simulink model "Galvo_sys_Cdisc_Pcont_cc_nosub_GUT_v63_algebLoop_refMods_101114"  (R2013a)
settings: Solver=ode45  StartTime=0.0  StopTime=10e-3  FixedStep=FS  MaxStep=1e-4  RelTol=1e-3
PreLoadFcn:
  | vname=@(x) inputname(1);
  | paramCtrl=evalin('base','paramCtrl;');
  | I_LIM=str2num(paramCtrl.I_LIM);
  | Kbc=str2num(paramCtrl.Kbc);
  | FS=evalin('base','FS;');
InitFcn:
  | %%%%%%  set scope time range
  | T_STOP=str2num(get_param(gcs,'StopTime'));
  | if numel(T_STOP) > 1
  |    T_STOP=T_STOP(2);
  | else
  |    T_STOP=T_STOP(1);
  | end
  | T_STOP=num2str(T_STOP);
  | 
  | %%%%%%  set scope time range in system @init_callback_fct
  | T_STOP=num2str(str2num(get_param(gcs,'StopTime')));
  | 
  | childs = allchild(0);
  | sol=strfind(upper(get(allchild(0),'Tag')),'VIEWER_PARAMETERS');
  | 
  | if iscell(sol)
  |    ind=find(~cellfun(@isempty, strfind(upper(get(allchild(0),'Tag')),'VIEWER_PARAMETERS')));
  | else
  |    ind=sol;
  | end
  | %ind=find(~cellfun(@isempty, {strfind(upper(get(allchild(0),'Tag')),'VIEWER_PARAMETERS'),[]}))
  | if ~isempty(ind)
  |    for k=1:length(childs(ind))
  |       set_param(getfield(get(childs(ind(k)),'UserData'),'block'),'TimeRange',T_STOP);
  |       get_param(getfield(get(childs(ind(k)),'UserData'),'block'),'TimeRange');
  | %    set_param(getfield(get(childs(ind),'UserData'),'block'),'TimeRange',T_STOP);
  | %    get_param(getfield(get(childs(ind),'UserData'),'block'),'TimeRange');
  |    end
  | else
  |     warning(sprintf('VIEWER_PARAMETERS object not found\nOpen the config dialog by hand for the first sim start'))
  | end
StartFcn:
  | I_LIM=str2num(paramCtrl.I_LIM);
  | Kbc=str2num(paramCtrl.Kbc);
  | %FS=evalin('base','FS;');
values from neighbouring files (symbols this model uses):
  FB_EN = 1    [GalvoModel_v6_sys.m]    (also in Galvo_process_analyze.m = k-1; kompl_kreis_linmod_sensitiv.m)
  Lc = 170e-6    (= 0.00017)    [GalvoModel_v6_sys.m]    (also in Galvo_process_analyze.m)
  Rc = 1.5    [GalvoModel_v6_sys.m]    (also in Galvo_process_analyze.m; frequenzgang_nichtinvert_opamp_koblitz_eas.m = 1)
  Rsh = 0.003    [GalvoModel_v6_sys.m]    (also in Galvo_sys_proto_v13_OFFSETS_MODEL_PT1B_proc.m = 0.075; frequenzgang_nichtinvert_opamp_koblitz_eas.m = 0.015)
undefined symbols (not defined in the file or in its folder): JR, KBM, KFR, KMT, KTB
libraries: simulink x2, simulink_extras x1, dspsigops x1
settings Model: BufferReuse=off  Creator=mainster  LastModifiedBy=mainster
settings SolverCC: AutoInsertRateTranBlk=on
settings DataIOCC: LimitDataPoints=off  SaveOutput=off  SaveTime=off
settings OptimizationCC: BlockReduction=off  OptimizeBlockIOStorage=off  BufferReuse=off  ExpressionFolding=off  LocalBlockOutputs=off
settings ModelReferenceCC: ModelReferenceNumInstancesAllowed=Single  ModelReferenceMinAlgLoopOccurrences=on

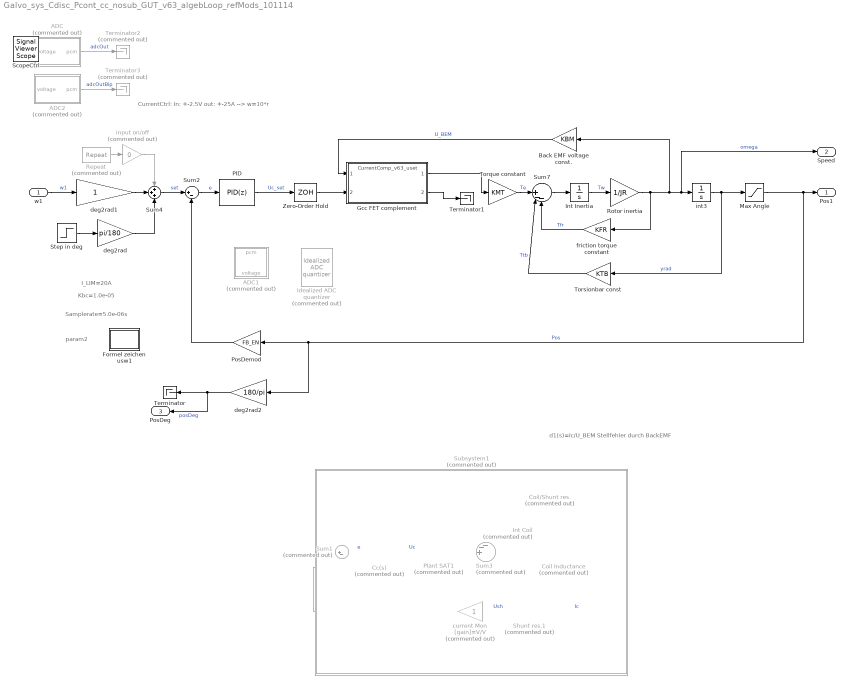
== system Galvo_sys_Cdisc_Pcont_cc_nosub_GUT_v63_algebLoop_refMods_101114 ==
  note: I_LIM=20A
  note: Kbc=1.0e-05
  note: Samplerate=5.0e-06s
  note: param2
  note: CurrentCtrl:
      | In:		+-2.5V
      | out: 	+-25A
      | --> w=10*r
  note: d1(s)=Ic/U_BEM
      | Stellfehler durch BackEMF
  w1 : Inport
  ADC : Subsystem  Commented=on
      mask Display: fprintf('ADC\n4-bit\n0-3V');
  ADC1 : Subsystem  Commented=on  mask{bypass=on}
      mask prompts: bypass "bypass adc"
      mask Callback bypass: %Simulink.Block.eval([gcb '/switch']);
      mask Display:
      | %fprintf('ADC\nGain=%s\n=%i',...
      | %    get_param([gcb '/scale'], 'Gain'),...
      | %    eval( get_param([gcb '/scale'], 'Gain') ));
      | if bypass
      |     color('red')
      |     fprintf('bypass\nADC')
      | else
      |     color('black')
      |     fprintf('ADC')
      | end
  ADC2 : Subsystem  Commented=on
      mask Display: fprintf('ADC\n4-bit\n-3...+3V');
  Back EMF voltage const. : Gain  Gain=KBM
  Cc(s) : simulink/Continuous/PID Controller  Commented=on  Controller=P  TimeDomain=Continuous-time  SampleTime=-1  IntegratorMethod=Forward Euler  FilterMethod=Forward Euler  Form=Ideal  P=18.7463154861029  I=14078.2261040339  D=0  N=100  InitialConditionSource=internal  InitialConditionForIntegrator=0  InitialConditionForFilter=0  ExternalReset=none  LimitOutput=off  UpperSaturationLimit=inf  LowerSaturationLimit=-inf  LinearizeAsGain=on  AntiWindupMode=none  Kb=1  TrackingMode=off  Kt=1  PParamMin=[]  PParamMax=[]  IParamMin=[]  IParamMax=[]  DParamMin=[]  DParamMax=[]  NParamMin=[]  NParamMax=[]  KbParamMin=[]  KbParamMax=[]  KtParamMin=[]  KtParamMax=[]  POutMin=[]  POutMax=[]  IOutMin=[]  IOutMax=[]  DOutMin=[]  DOutMax=[]  NOutMin=[]  NOutMax=[]  KbOutMin=[]  KbOutMax=[]  KtOutMin=[]  KtOutMax=[]  IntegratorOutMin=[]  IntegratorOutMax=[]  FilterOutMin=[]  FilterOutMax=[]  SumOutMin=[]  SumOutMax=[]  SumI1OutMin=[]  SumI1OutMax=[]  SumI2OutMin=[]  SumI2OutMax=[]  SumI3OutMin=[]  SumI3OutMax=[]  SumDOutMin=[]  SumDOutMax=[]  SaturationOutMin=[]  SaturationOutMax=[]  IntegratorContinuousStateAttributes=''  IntegratorStateMustResolveToSignalObject=off  IntegratorRTWStateStorageClass=Auto  FilterContinuousStateAttributes=''  FilterStateMustResolveToSignalObject=off  FilterRTWStateStorageClass=Auto
  Coil Inductance : Gain  Commented=on  Gain=1/Lc
  Coil/Shunt res. : Gain  Commented=on  Gain=Rc+Rsh
  Formel zeichen usw1 : Subsystem
  Gcc FET complement : ModelReference  ModelNameDialog=CurrentComp_v63_uset.slx  SimulationMode=Normal  Variant=on  ModelReferenceVersion=1.112  CopyOfModelName=CurrentComp_v63_uset.slx  DefaultDataLogging=on
      mask Display:
      | str=sprintf('%s',get(gcbh,'ModelName'));
      | port_label('input', 1, 'U_{BEM}','texmode','on')
      | port_label('input', 2, 'I/U_{Set}','texmode','on')
      | port_label('output', 1, 'I_{Coil}','texmode','on')
      | port_label('output', 2, 'U_{Coil}','texmode','on')
      | %text(.05,.98,['{\fontsize{12}\it\bf' strrep(str,'_',' ') '}'],'horizontalAlignment','left','verticalAlignment','top','texmode','on')
      | text(.5,0.95,['{\fontsize{12}\it\bfG_{cc}(s)}'],'horizontalAlignment','center','verticalAlignment','top','texmode','on')
      | text(.5,0.65,['{\fontsize{14}\it\bfFET v1}'],'horizontalAlignment','center','verticalAlignment','top','texmode','on')
      | %text(.15,.05,['{\fontsize{10}\itmechanics}'],'horizontalAlignment','left','verticalAlignment','bottom','texmode','on')
  Idealized ADC quantizer : simulink_extras/Additional Discrete/Idealized ADC quantizer  Commented=on  NumberOfConverterBits=16  Vmin=-0.5  Vmax=0.5  OutputDataType=int16  OutputNegativeValues=on
  Int Coil : Integrator  Commented=on
  Int Inertia : Integrator
  Max Angle : Saturate  UpperLimit=20*pi/180  LowerLimit=-20*pi/180
      settings: AttributesFormatString=Max=%<UpperLimit>\nMin=%<LowerLimit>
  PID : simulink/Continuous/PID Controller  Controller=PID  TimeDomain=Discrete-time  SampleTime=FS  IntegratorMethod=Forward Euler  FilterMethod=Forward Euler  Form=Parallel  P=0.655816611321994  I=1.94996274175201  D=0.00199528604043407  N=726.725522130778  InitialConditionSource=internal  InitialConditionForIntegrator=0  InitialConditionForFilter=0  ExternalReset=none  IgnoreLimit=on  LimitOutput=on  UpperSaturationLimit=30  LowerSaturationLimit=-30  LinearizeAsGain=off  AntiWindupMode=clamping  Kb=0.1  TrackingMode=off  Kt=0  PParamMin=[]  PParamMax=[]  IParamMin=[]  IParamMax=[]  DParamMin=[]  DParamMax=[]  NParamMin=[]  NParamMax=[]  KbParamMin=[]  KbParamMax=[]  KtParamMin=[]  KtParamMax=[]  POutMin=[]  POutMax=[]  IOutMin=[]  IOutMax=[]  DOutMin=[]  DOutMax=[]  NOutMin=[]  NOutMax=[]  KbOutMin=[]  KbOutMax=[]  KtOutMin=[]  KtOutMax=[]  IntegratorOutMin=[]  IntegratorOutMax=[]  FilterOutMin=[]  FilterOutMax=[]  SumOutMin=[]  SumOutMax=[]  SumI1OutMin=[]  SumI1OutMax=[]  SumI2OutMin=[]  SumI2OutMax=[]  SumI3OutMin=[]  SumI3OutMax=[]  SumDOutMin=[]  SumDOutMax=[]  SaturationOutMin=[]  SaturationOutMax=[]  IntegratorContinuousStateAttributes=''  IntegratorStateMustResolveToSignalObject=off  IntegratorRTWStateStorageClass=Auto  FilterContinuousStateAttributes=''  FilterStateMustResolveToSignalObject=off  FilterRTWStateStorageClass=Auto
  Plant SAT1 : Saturate  Commented=on  UpperLimit=30  LowerLimit=-30
      settings: AttributesFormatString=U_lim=+-%<UpperLimit>V
  PosDemod : Gain  Gain=FB_EN
  Repeat : dspsigops/Repeat  Commented=on  N=length(str2num(get_param([gcs '/Sequence Stair'], 'OutValues')))  InputProcessing=Columns as channels (frame based)  RateOptions=Allow multirate processing  ic=0  mode=Unused parameter value
  Rotor inertia : Gain  Gain=1/JR
  Shunt res.1 : Gain  Commented=on
  Step in deg : Step  Time=1e-3  After=5  SampleTime=FS  ZeroCross=off
      settings: AttributesFormatString=Ampl.: %<After>\ntime:%<Time>
  Subsystem1 : Subsystem  Commented=on
      mask Display: text(.05,.05,['{\fontsize{13}\it\bfCurrent comp}'],'horizontalAlignment','left','verticalAlignment','bottom','texmode','on')
  Sum1 : Sum  Commented=on  Inputs=|+-
  Sum2 : Sum  Inputs=|+-
  Sum3 : Sum  Commented=on  Inputs=--+||
  Sum4 : Sum  Inputs=+++  SampleTime=FS
  Sum7 : Sum  Inputs=||+--
  Terminator : Terminator
  Terminator1 : Terminator
  Terminator2 : Terminator  Commented=on
  Terminator3 : Terminator  Commented=on
  Torque constant : Gain  Gain=KMT  SampleTime=0
  Torsionbar const : Gain  Gain=KTB
  Zero-Order Hold : ZeroOrderHold  SampleTime=-1
  current Mon [gain]=V/V : Gain  Commented=on
  deg2rad : Gain  Gain=pi/180  SampleTime=FS
  deg2rad1 : Gain  SampleTime=FS
  deg2rad2 : Gain  Gain=180/pi
  friction torque constant : Gain  Gain=KFR
  input on/off : Gain  Commented=on  Gain=0  SampleTime=FS
  int3 : Integrator
  Pos1 : Outport
  Speed : Outport  Port=2
  PosDeg : Outport  Port=3
  ScopeCtrl : SignalViewerScope  IOType=viewer  NumInputPorts=5  LegendLocations=|  RefreshTime=0.033391
      | 0.82124     0.92196     0.12993    0.037382
      | 0.78898     0.74948     0.16219    0.020986
      |       0           0           0           0
      | 0.79973     0.37067     0.15143    0.020986
      | 0.73522     0.16435     0.21595    0.037382
      settings: ShowLegends=on  TimeRange=0.005  YMin=0~-1.2e-05~-1~-0.0005~0  YMax=0.09~4e-06~3~0.0005~5
  wires:
  w1/1 -> deg2rad1/1  "w1"
  Repeat/1 -> input on/off/1
  Sum2/1 -> PID/1  "e"
  Sum4/1 -> Sum2/1  "set"
  Step in deg/1 -> deg2rad/1
  input on/off/1 -> Sum4/1
  deg2rad/1 -> Sum4/3
  int3/1 -> Max Angle/1, Torsionbar const/1  "yrad"
  Int Inertia/1 -> Rotor inertia/1  "Tw"
  Sum7/1 -> Int Inertia/1
  Rotor inertia/1 -> Speed/1, int3/1, Back EMF voltage const./1, friction torque constant/1  "omega"
  friction torque constant/1 -> Sum7/3  "Tfr"
  Max Angle/1 -> deg2rad2/1, PosDemod/1, Pos1/1  "Pos"
  Torque constant/1 -> Sum7/1  "Te"
  Torsionbar const/1 -> Sum7/2  "Ttb"
  PID/1 -> Zero-Order Hold/1  "Uc_set"
  deg2rad2/1 -> PosDeg/1, Terminator/1  "posDeg"
  deg2rad1/1 -> Sum4/2
  Sum1/1 -> Cc(s)/1  "e"
  Coil Inductance/1 -> Shunt res.1/1, Coil/Shunt res./1  "Ic"
  Coil/Shunt res./1 -> Sum3/1
  Sum3/1 -> Int Coil/1
  Int Coil/1 -> Coil Inductance/1
  Cc(s)/1 -> Plant SAT1/1  "Uc"
  Shunt res.1/1 -> current Mon [gain]=V/V/1  "Ush"
  current Mon [gain]=V/V/1 -> Sum1/2
  Plant SAT1/1 -> Sum3/3
  Back EMF voltage const./1 -> Gcc FET complement/1  "U_BEM"
  Zero-Order Hold/1 -> Gcc FET complement/2
  Gcc FET complement/1 -> Torque constant/1
  Gcc FET complement/2 -> Terminator1/1
  PosDemod/1 -> Sum2/2
  ADC/1(pcm) -> Terminator2/1  "adcOut"
  ADC2/1(pcm) -> Terminator3/1  "adcOutBip"

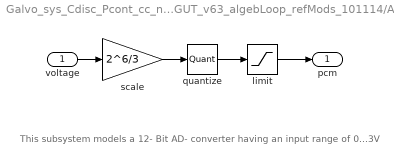
== system Galvo_sys_Cdisc_Pcont_cc_nosub_GUT_v63_algebLoop_refMods_101114/ADC ==
  note: This subsystem models a 12- Bit AD- converter
      | having an input  range of 0...3V
  voltage : Inport
  limit : Saturate  UpperLimit=2^12  LowerLimit=0
  quantize : Quantizer
  scale : Gain  Gain=2^6/3  SaturateOnIntegerOverflow=on  OutDataTypeStr=Inherit: Same as input  ParamDataTypeStr=Inherit: Same as input
  pcm : Outport
  wires:
  limit/1 -> pcm/1
  scale/1 -> quantize/1
  quantize/1 -> limit/1
  voltage/1 -> scale/1

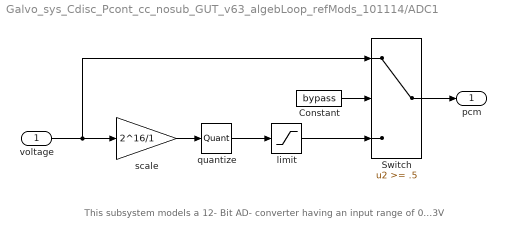
== system Galvo_sys_Cdisc_Pcont_cc_nosub_GUT_v63_algebLoop_refMods_101114/ADC1 ==
  note: This subsystem models a 12- Bit AD- converter
      | having an input  range of 0...3V
  voltage : Inport
  Constant : Constant  Value=bypass
  Switch : Switch  Threshold=.5
  limit : Saturate  UpperLimit=2^15-1  LowerLimit=-2^15
  quantize : Quantizer
  scale : Gain  Gain=2^16/1  SaturateOnIntegerOverflow=on  OutDataTypeStr=Inherit: Same as input  ParamDataTypeStr=Inherit: Same as input
  pcm : Outport
  wires:
  limit/1 -> Switch/3
  scale/1 -> quantize/1
  quantize/1 -> limit/1
  voltage/1 -> Switch/1, scale/1
  Constant/1 -> Switch/2
  Switch/1 -> pcm/1

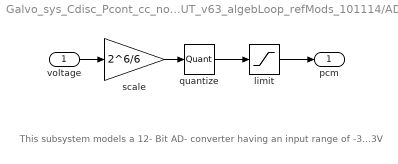
== system Galvo_sys_Cdisc_Pcont_cc_nosub_GUT_v63_algebLoop_refMods_101114/ADC2 ==
  note: This subsystem models a 12- Bit AD- converter
      | having an input  range of -3...3V
  voltage : Inport
  limit : Saturate  UpperLimit=2^5-1  LowerLimit=-2^5
  quantize : Quantizer
  scale : Gain  Gain=2^6/6  SaturateOnIntegerOverflow=on  OutDataTypeStr=Inherit: Same as input  ParamDataTypeStr=Inherit: Same as input
  pcm : Outport
  wires:
  limit/1 -> pcm/1
  scale/1 -> quantize/1
  quantize/1 -> limit/1
  voltage/1 -> scale/1

== system Galvo_sys_Cdisc_Pcont_cc_nosub_GUT_v63_algebLoop_refMods_101114/Formel zeichen usw1 ==
  note: Te: 		electrical torque, gen. by coils		[Nm]
      |  Ic: 			coil current							[A]
      |  Tfr:		rotor dynamic friction torque 		[Nm]
      |  Trb:		torsion bar torque					[Nm]
      |  Tw:		angular momentum				[Nm*s]
      |  w:			angular velocity 					[rad/s]
      |  yrad:		angular position 					[rad]
      |  ydeg:		angular position 					[°]
      |  Ucci:		current controller input				[V]
      |  Ucco:		current controller output			[V]
      |  Ush:		shunt voltage						[V]
  note: L_{c  }	coil inductance 							[H]
      |  R_{c  }	coil resistance							[\Omega]
      |  R_{SH }	current shunt resistance				[\Omega]
      |  J_{R  }	rotor inertia 							[kg*m²]
      |  K_{TB }	torsion bar torque const. 			[Nm/rad]
      |  K_{BM }	back EMF const.							[V*s/rad]
      |  K_{FR }	rotor dyn. friction torque const.	[Nm*s/rad]
      |  K_{MT }	el. magnetic torque const.			[Nm/A]
  note: balance of force: 	Te=Ttb+Tfr
      | 					Te - (Ttb+Tfr)=0  ->  no movement
      |
      |  integrate( 1 Nm )dt = 1 Nm*s
      |  (Nm*s)(kg*m²)⁻¹ = (N*s/kg)*m⁻¹ = m/(s*m) = rad

== system Galvo_sys_Cdisc_Pcont_cc_nosub_GUT_v63_algebLoop_refMods_101114/Subsystem1 ==
